simulink model "Ideal_Control_System"  (R2025b)
settings: Solver=FixedStepAuto  StartTime=0.0  StopTime=tspan  FixedStep=dt_sim  RelTol=rel_tol  AbsTol=abs_tol
undefined symbols (not defined in the file): battery_voltage, mission_file
settings Model: Creator=koryh  LastModifiedBy=koryh

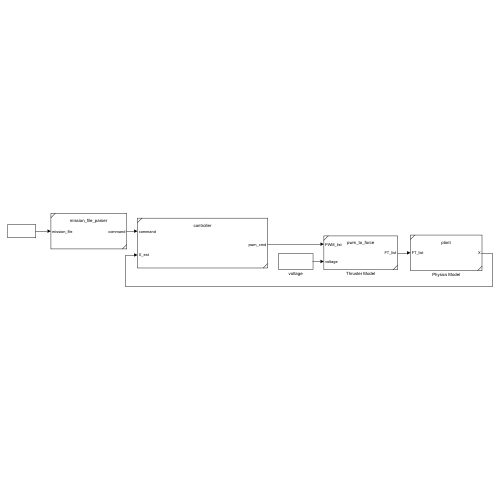
[thumbnail: Simulink's stored preview of the top-level diagram]
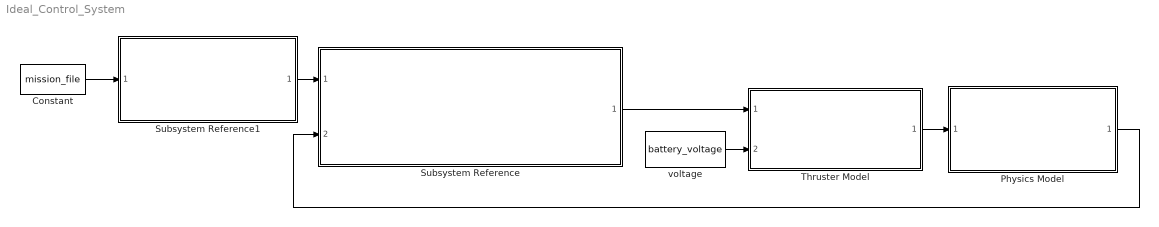
== system Ideal_Control_System ==
  Constant : Constant  Value=mission_file
  Physics Model : Subsystem  ReferencedSubsystem=plant
  Subsystem Reference : Subsystem  ReferencedSubsystem=controller
  Subsystem Reference1 : Subsystem  ReferencedSubsystem=mission_file_parser
  Thruster Model : Subsystem  ReferencedSubsystem=pwm_to_force
  voltage : Constant  Value=battery_voltage
  wires:
  Thruster Model/1 -> Physics Model/1
  voltage/1 -> Thruster Model/2
  Subsystem Reference/1 -> Thruster Model/1
  Subsystem Reference1/1 -> Subsystem Reference/1
  Constant/1 -> Subsystem Reference1/1
  Physics Model/1 -> Subsystem Reference/2
